simulink model "IEEE_39_IBR_Simplified"  (R2023b)
settings: Solver=FixedStepAuto  StartTime=0  StopTime=20  FixedStep=Ts  MaxStep=1/60  RelTol=1e-3  AbsTol=1e-2  EnableMultiTasking=on
PreLoadFcn:
  | NE39bus_data;
  | PSSMODEL=1;
  | LPSS=0;
  | WAPSS=0;
  | WAPSS2=0;
values from neighbouring files (symbols this model uses):
  Dt = 0    [SG_para.m]
  dw0_sm = 0    [SG_para.m]
  Emax = 1    [SG_para.m]
  Emin = 0.5    [SG_para.m]
  Fg = [0.1,0.1,0.1]    [SG_para.m]
  fn_sm = 60*ones(1,10)    [SG_para.m]
  H_sm = [5,3.03,3.58,2.86,2.6,3.48,2.64,2.43,3.45,4.2]*10    [SG_para.m]
  ia0_sm = 0.75*0    (= 0)    [SG_para.m]
  ib0_sm = 0.75*0    (= 0)    [SG_para.m]
  ic0_sm = 0.75*0    (= 0)    [SG_para.m]
  Kd_sm = 6*ones(1,10)    [SG_para.m]
  Ke = 200    [SG_para.m]
  Kg = [0.95,0.95,0.95]    [SG_para.m]
  Ks = 2    [SG_para.m]
  line = [     1	2	0.0035	0.0411	0.6987	0	100	345 ... (first row only)    [SG_para.m]
  p = 1    [SG_para.m]
  pha0_sm = -24.95*0    (= 0)    [SG_para.m]
  phb0_sm = -144.94*0    (= 0)    [SG_para.m]
  phc0_sm = 95.05*0    (= 0)    [SG_para.m]
  Pn_sm = [1000,1000,1000,1000,1000,1000,1000,1000,1000,1000]    [SG_para.m]
  Pref_sm = [1000 520.81 650 632 508 650 560 540 830 250]./Pn_sm    [SG_para.m]
  R = 1e-3    (= 0.001)    [SG_para.m]
  Rg = [0.05,0.05,0.05]    [SG_para.m]
  rs = 2.8544e-3    (= 0.0028544)    [SG_para.m]
  s = 1    [SG_para.m]
  s1 = 10    [SG_para.m]
  T1 = 0.05    [SG_para.m]
  T2 = 0.5    [SG_para.m]
  T3 = 0.5    [SG_para.m]
  Te = 0.05    [SG_para.m]
  Tfa = 3    [SG_para.m]
  Tfb = 10    [SG_para.m]
  Tg = [10,10,10]    [SG_para.m]
  theta0_sm = -94.3*0    (= 0)    [SG_para.m]
  Ts = 5e-5    (= 5e-05)    [SG_para.m]
  Ts1 = 0.18    [SG_para.m]
  Ts2 = 2    [SG_para.m]
  Ts3 = 5    [SG_para.m]
  Ts4 = 10    [SG_para.m]
  Ts5 = 15    [SG_para.m]
  Un_sm = [345,22,22,22,22,22,22,22,345,22]    [SG_para.m]
  Vmax = inf    [SG_para.m]
  Vmin = 0    [SG_para.m]
  Vref_sm = 1*ones(1,10)    [SG_para.m]
  xd = xd_t    (= 0.296)    [SG_para.m]
undefined symbols (not defined in the file or in its folder): D1, D11, Delta, Ka, Kf, Ta, Tf
libraries: spsThreePhaseVIMeasurementLib x41, spsThreePhaseFaultLib x39, spsThreePhaseSeriesRLCBranchLib x36, spsThreePhaseParallelRLCLoadLib x20, spsThreePhaseTransformerTwoWindingsLib x13, spsSimplifiedSynchronousMachinepuUnitsLib x10, spsLoadFlowBusLib x10, Inverter_based_Resources_IBRs x10, spsThreePhaseBreakerLib x2, spsSequenceAnalyzerLib x2, spsMultimeterLib x1, eePowerMeasurement x1
(part 1 of 5)
settings Model: SimulationMode=accelerator  Creator=Innocent  LastModifiedBy=qholmes
settings SolverCC: AutoScaleAbsTol=off  ZeroCrossAlgorithm=Adaptive  AlgebraicLoopSolver=TrustRegion
settings DataIOCC: SaveFormat=Array  SignalLoggingSaveFormat=ModelDataLogs  SaveOutput=off  SaveTime=off  ReturnWorkspaceOutputs=off
settings OptimizationCC: BlockReduction=off  BooleanDataType=off  ExpressionDepthLimit=2147483647  InitFltsAndDblsToZero=on  LifeSpan=inf
settings DebuggingCC: SaveWithParameterizedLinksMsg=none  UnderspecifiedInitializationDetection=Classic  MergeDetectMultiDrivingBlocksExec=none  SignalResolutionControl=TryResolveAllWithWarning  MaxConsecutiveZCsMsg=none  SolverPrmCheckMsg=warning  MultiTaskDSMMsg=warning  MultiTaskCondExecSysMsg=none  FcnCallInpInsideContextMsg=warning  StateNameClashWarn=warning  SFUnexpectedBacktrackingDiag=warning  SFNoUnconditionalDefaultTransitionDiag=warning  SFExecutionAtInitializationDiag=none  ArithmeticOperatorsInVariantConditions=warning
settings HardwareCC: ProdBitPerPointer=32  ProdBitPerSizeT=32  ProdBitPerPtrDiffT=32  ProdLargestAtomicFloat=None  ProdIntDivRoundTo=Undefined  ProdEndianess=Unspecified  ProdWordSize=32  ProdHWDeviceType=32-bit Generic
settings ModelReferenceCC: EnableRefExpFcnMdlSchedulingChecks=on  PropagateSignalLabelsOutOfModel=off
settings SFSimCC: SimUseLocalCustomCode=off  CustomCodeUndefinedFunction=UseInterfaceOnly
settings RTWCC: RTWUseLocalCustomCode=off  DLArmComputeVersion=19.05
settings CodeAppCC: StateflowObjectComments=on
settings GRTTargetCC: TargetFcnLib=ansi_tfl_tmw.mat  TargetLangStandard=C89/C90 (ANSI)  CombineOutputUpdateFcns=off  GRTInterface=on
settings ConfigComp: CovMetricSettings=dw  CovSaveCumulativeToWorkspaceVar=on  CovSaveSingleToWorkspaceVar=on  CovExternalEMLEnable=off
settings SimscapeCC: SimscapeNormalizeSystem=off

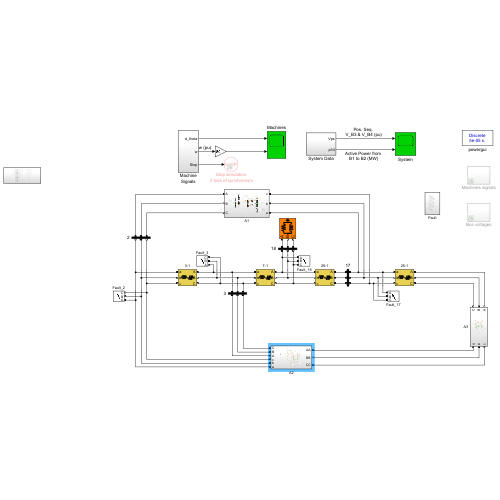
[thumbnail: Simulink's stored preview of the top-level diagram]
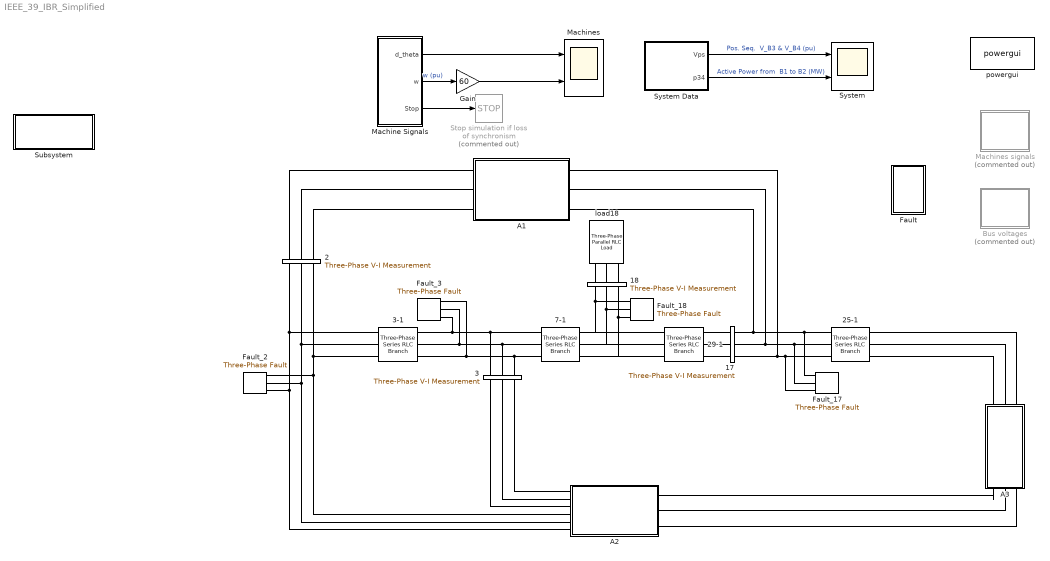
== system IEEE_39_IBR_Simplified ==
  17 : spsThreePhaseVIMeasurementLib/Three-Phase V-I Measurement  VoltageMeasurement=phase-to-phase  SetLabelV=on  LabelV=Vabc_17  Vpu=off  VpuLL=on  CurrentMeasurement=no  SetLabelI=on  LabelI=Iabc_B2  Ipu=off  Pbase=100e6  Vbase=Bus(17,2)*1e3  OutputType=Complex  PhasorSimulation=off  PSBequivalent=0
  18 : spsThreePhaseVIMeasurementLib/Three-Phase V-I Measurement  VoltageMeasurement=phase-to-phase  SetLabelV=on  LabelV=Vabc_18  Vpu=off  VpuLL=on  CurrentMeasurement=no  SetLabelI=on  LabelI=Iabc_B2  Ipu=off  Pbase=100e6  Vbase=Bus(18,2)*1e3  OutputType=Complex  PhasorSimulation=off  PSBequivalent=0
  2 : spsThreePhaseVIMeasurementLib/Three-Phase V-I Measurement  VoltageMeasurement=phase-to-phase  SetLabelV=on  LabelV=Vabc_2  Vpu=off  VpuLL=on  CurrentMeasurement=no  SetLabelI=on  LabelI=Iabc_B2  Ipu=off  Pbase=100e6  Vbase=Bus(2,2)*1e3  OutputType=Complex  PhasorSimulation=off  PSBequivalent=0
  25-1 : spsThreePhaseSeriesRLCBranchLib/Three-Phase Series RLC Branch  LConnTagsString=A|B|C  RConnTagsString=A|B|C  BranchType=RL  Resistance=line(25,3)  Inductance=line(25,4)  Capacitance=1e-6  Measurements=None
  29-1 : spsThreePhaseSeriesRLCBranchLib/Three-Phase Series RLC Branch  LConnTagsString=A|B|C  RConnTagsString=A|B|C  BranchType=RL  Resistance=line(29,3)  Inductance=line(29,4)  Capacitance=1e-6  Measurements=None
  3 : spsThreePhaseVIMeasurementLib/Three-Phase V-I Measurement  VoltageMeasurement=phase-to-phase  SetLabelV=on  LabelV=Vabc_B3  Vpu=off  VpuLL=on  CurrentMeasurement=yes  SetLabelI=on  LabelI=Iabc_B3  Ipu=off  Pbase=100e6  Vbase=Bus(3,2)*1e3  OutputType=Complex  PhasorSimulation=off  PSBequivalent=0
  3-1 : spsThreePhaseSeriesRLCBranchLib/Three-Phase Series RLC Branch  LConnTagsString=A|B|C  RConnTagsString=A|B|C  BranchType=RL  Resistance=line(3,3)  Inductance=line(3,4)  Capacitance=1e-6  Measurements=None
  7-1 : spsThreePhaseSeriesRLCBranchLib/Three-Phase Series RLC Branch  LConnTagsString=A|B|C  RConnTagsString=A|B|C  BranchType=RL  Resistance=line(7,3)  Inductance=line(7,4)  Capacitance=1e-6  Measurements=None
  A1 : Subsystem
  A2 : Subsystem
  A3 : Subsystem
  Bus voltages : Subsystem  Commented=on
  Fault : Subsystem
  Fault_17 : spsThreePhaseFaultLib/Three-Phase Fault  InitialStates=0  FaultA=on  FaultB=on  FaultC=on  GroundFault=on  SwitchTimes="[t(17)+1/60  t(17)+5/60]"  External=off  SwitchStatus=NaN  FaultResistance=0.001  GroundResistance=0.01  SnubberResistance=1e6  SnubberCapacitance=inf  Measurements=Fault voltages and currents
  Fault_18 : spsThreePhaseFaultLib/Three-Phase Fault  InitialStates=0  FaultA=on  FaultB=on  FaultC=on  GroundFault=on  SwitchTimes="[t(18)+1/60  t(18)+5/60]"  External=off  SwitchStatus=NaN  FaultResistance=0.001  GroundResistance=0.01  SnubberResistance=1e6  SnubberCapacitance=inf  Measurements=Fault voltages and currents
  Fault_2 : spsThreePhaseFaultLib/Three-Phase Fault  InitialStates=0  FaultA=on  FaultB=on  FaultC=on  GroundFault=on  SwitchTimes="[t(2)+1/60  t(2)+5/60]"  External=off  SwitchStatus=NaN  FaultResistance=0.001  GroundResistance=0.01  SnubberResistance=1e6  SnubberCapacitance=inf  Measurements=Fault voltages and currents
  Fault_3 : spsThreePhaseFaultLib/Three-Phase Fault  InitialStates=0  FaultA=on  FaultB=on  FaultC=on  GroundFault=on  SwitchTimes="[t(3)+1/60  t(3)+5/60]"  External=off  SwitchStatus=NaN  FaultResistance=0.001  GroundResistance=0.01  SnubberResistance=1e6  SnubberCapacitance=inf  Measurements=Fault voltages and currents
  Gain : Gain  Gain=60
  Machine Signals : Subsystem
  Machines : Scope  NumInputPorts=2
  Machines signals : Subsystem  Commented=on
  Stop simulation if loss of synchronism : Stop  Commented=on
  Subsystem : Subsystem
  System : Scope  NumInputPorts=2
  System Data : Subsystem
  load18 : spsThreePhaseParallelRLCLoadLib/Three-Phase Parallel RLC Load  LConnTagsString=A|B|C  Configuration=Y (grounded)  NominalVoltage=(345000)*0.991132  Vabc=[1e3 1e3 1e3]  Vabcp=[1e3 1e3 1e3]  NominalFrequency=60  UnbalancedPower=off  ActivePower=158e6  InductivePower=30e6  CapacitivePower=0  Pabc=[10e3 9e3 11e3]  QLabc=[100 90 110]  QCabc=[100 90 110]  Pabcp=[10e3 9e3 11e3]  QLabcp=[100 90 110]  QCabcp=[100 90 110]  Measurements=None  LoadType=constant PQ
  powergui : sps_lib/powergui  Priority=2  SimulationMode=Discrete  SampleTime=Ts  frequency=60  Iterations=50  frequencyindice=0  Pbase=100e6  ErrMax=0.0001  UnitsV=kV  UnitsW=MW  buscounter=0  FunctionMessages=off  echomessages=off  EnableUseOfTLC=off  CurrentSourceSwitches=off  DisableSnubberDevices=off  DisableRonSwitches=off  DisableVfSwitches=off  DisplayEquations=off  AutomaticDiscreteSolvers=off  SolverType=Tustin/Backward Euler (TBE)  Interpol=off  ExternalGateDelay=off  methode=off  Ts=100  x0status=blocks  SPID=off  SwTol=0  HookPort=off  NonlinearTolerance=1e-4  nMaxIteration=100  ContinueOnMaxIteration=off  RestoreLinks=warning  ResistiveCurrentMeasurement=off  Frange=logspace(0,3,50)  Ylog=off  Xlog=off  ShowGrid=off  save=off  variable=ZData  structure=0  ZoomFFT=on  StartTime=0.0  cycles=1  DisplayStyle=1  fundamental=60  FreqAxis=off  MaxFrequency=1000  frequencyindicesteady=1  RmsSteady=1  display=off
  wires:
  Machine Signals/2(w) -> Gain/1  "w (pu)"
  Machine Signals/3(Stop) -> Stop simulation if loss of synchronism/1
  Machine Signals/1(d_theta) -> Machines/1
  System Data/1(Vps) -> System/1  "Pos. Seq.  V_B3 & V_B4 (pu)"
  System Data/2(p34) -> System/2  "Active Power from  B1 to B2 (MW)"
  Gain/1 -> Machines/2
  connections:
  29-1/LConn1 -- 17/RConn1
  29-1/LConn2 -- 17/RConn2
  29-1/LConn3 -- 17/RConn3
  load18/LConn1 -- 18/LConn1
  load18/LConn2 -- 18/LConn2
  load18/LConn3 -- 18/LConn3
  3/LConn1 -- 7-1/RConn1 -- 3-1/LConn1 -- Fault_3/LConn1
  Fault_3/LConn2 -- 3-1/LConn2 -- 7-1/RConn2 -- 3/LConn2
  Fault_3/LConn3 -- 3-1/LConn3 -- 7-1/RConn3 -- 3/LConn3
  Fault_2/LConn3 -- A2/LConn4 -- 3-1/RConn3 -- 2/RConn3
  29-1/RConn1 -- 7-1/LConn1 -- Fault_18/LConn1 -- 18/RConn1
  29-1/RConn2 -- 7-1/LConn2 -- Fault_18/LConn2 -- 18/RConn2
  29-1/RConn3 -- 7-1/LConn3 -- Fault_18/LConn3 -- 18/RConn3
  Fault_17/LConn2 -- 25-1/RConn2 -- A1/RConn2 -- 17/LConn2
  Fault_17/LConn3 -- 25-1/RConn3 -- A1/RConn1 -- 17/LConn3
  Fault_17/LConn1 -- 25-1/RConn1 -- A1/RConn3 -- 17/LConn1
  A1/LConn1 -- 2/LConn1
  A1/LConn2 -- 2/LConn2
  A1/LConn3 -- 2/LConn3
  25-1/LConn1 -- A3/LConn3
  25-1/LConn2 -- A3/LConn2
  25-1/LConn3 -- A3/LConn1
  Fault_2/LConn1 -- A2/LConn6 -- 3-1/RConn1 -- 2/RConn1
  Fault_2/LConn2 -- A2/LConn5 -- 3-1/RConn2 -- 2/RConn2
  3/RConn1 -- A2/LConn3
  3/RConn2 -- A2/LConn2
  A2/LConn1 -- 3/RConn3
  A3/RConn1 -- A2/RConn1
  A3/RConn2 -- A2/RConn2
  A3/RConn3 -- A2/RConn3

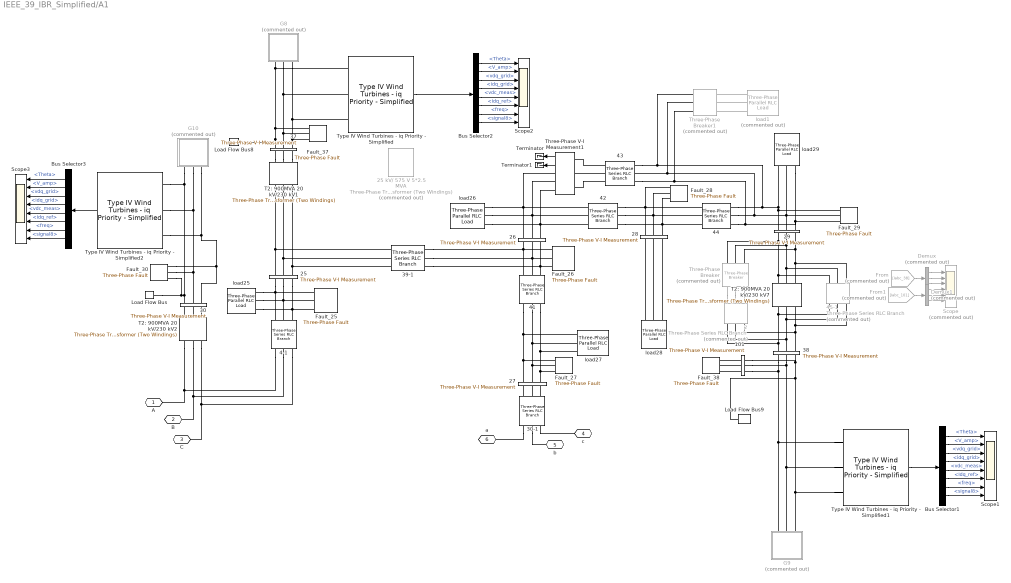
== system IEEE_39_IBR_Simplified/A1 ==
  101 : spsThreePhaseVIMeasurementLib/Three-Phase V-I Measurement  VoltageMeasurement=phase-to-phase  SetLabelV=on  LabelV=Vabc_101  Vpu=off  VpuLL=on  CurrentMeasurement=yes  SetLabelI=on  LabelI=Iabc_101  Ipu=off  Pbase=100e6  Vbase=345*1e3  OutputType=Complex  PhasorSimulation=off  PSBequivalent=0
  2 : spsThreePhaseSeriesRLCBranchLib/Three-Phase Series RLC Branch  Commented=on  LConnTagsString=A|B|C  RConnTagsString=A|B|C  BranchType=RL  Resistance=line(45,3)  Inductance=line(45,4)  Capacitance=1e-6  Measurements=None
  25 : spsThreePhaseVIMeasurementLib/Three-Phase V-I Measurement  VoltageMeasurement=phase-to-phase  SetLabelV=on  LabelV=Vabc_25  Vpu=off  VpuLL=on  CurrentMeasurement=no  SetLabelI=on  LabelI=Iabc_B2  Ipu=off  Pbase=100e6  Vbase=Bus(25,2)*1e3  OutputType=Complex  PhasorSimulation=off  PSBequivalent=0
  25 kV/ 575 V 5*2.5 MVA : spsThreePhaseTransformerTwoWindingsLib/Three-Phase Transformer (Two Windings)  Commented=on  Winding1Connection=Delta (D11)  Winding2Connection=Yg  CoreType=Three single-phase transformers  SetSaturation=off  Hysteresis=off  DataFile='hysteresis'  SetInitialFlux=off  Measurements=None  UNITS=pu  NominalPower="[2.5e6*400  60]"  Winding1=[22e3 , 0.025/30 , 0.025]  Winding2=[ 575, 0.025/30 , 0.025]  Rm=500  Lm=inf  L0=0.5  Saturation=[ 0,0 ; 0.0024,1.2 ; 1.0,1.52 ]  InitialFluxes=[ 0.8 , -0.8 , 0.7 ]  BreakLoop=off  DiscreteSolver=Trapezoidal iterative  DataType=off  TransfoNumber=0
  26 : spsThreePhaseVIMeasurementLib/Three-Phase V-I Measurement  VoltageMeasurement=phase-to-phase  SetLabelV=on  LabelV=Vabc_26  Vpu=off  VpuLL=on  CurrentMeasurement=no  SetLabelI=on  LabelI=Iabc_B2  Ipu=off  Pbase=100e6  Vbase=Bus(26,2)*1e3  OutputType=Complex  PhasorSimulation=off  PSBequivalent=0
  27 : spsThreePhaseVIMeasurementLib/Three-Phase V-I Measurement  VoltageMeasurement=phase-to-phase  SetLabelV=on  LabelV=Vabc_27  Vpu=off  VpuLL=on  CurrentMeasurement=no  SetLabelI=on  LabelI=Iabc_B2  Ipu=off  Pbase=100e6  Vbase=Bus(27,2)*1e3  OutputType=Complex  PhasorSimulation=off  PSBequivalent=0
  28 : spsThreePhaseVIMeasurementLib/Three-Phase V-I Measurement  VoltageMeasurement=phase-to-phase  SetLabelV=on  LabelV=Vabc_28  Vpu=off  VpuLL=on  CurrentMeasurement=no  SetLabelI=on  LabelI=Iabc_B2  Ipu=off  Pbase=100e6  Vbase=Bus(28,2)*1e3  OutputType=Complex  PhasorSimulation=off  PSBequivalent=0
  29 : spsThreePhaseVIMeasurementLib/Three-Phase V-I Measurement  VoltageMeasurement=phase-to-phase  SetLabelV=on  LabelV=Vabc_29  Vpu=off  VpuLL=on  CurrentMeasurement=no  SetLabelI=on  LabelI=Iabc_B2  Ipu=off  Pbase=100e6  Vbase=Bus(29,2)*1e3  OutputType=Complex  PhasorSimulation=off  PSBequivalent=0
  30 : spsThreePhaseVIMeasurementLib/Three-Phase V-I Measurement  VoltageMeasurement=phase-to-phase  SetLabelV=on  LabelV=Vabc_30  Vpu=off  VpuLL=on  CurrentMeasurement=no  SetLabelI=on  LabelI=Iabc_B2  Ipu=off  Pbase=100e6  Vbase=Bus(30,2)*1e3  OutputType=Complex  PhasorSimulation=off  PSBequivalent=0
  30-1 : spsThreePhaseSeriesRLCBranchLib/Three-Phase Series RLC Branch  LConnTagsString=A|B|C  RConnTagsString=A|B|C  BranchType=RL  Resistance=line(30,3)  Inductance=line(30,4)  Capacitance=1e-6  Measurements=None
  37 : spsThreePhaseVIMeasurementLib/Three-Phase V-I Measurement  VoltageMeasurement=phase-to-phase  SetLabelV=on  LabelV=Vabc_37  Vpu=off  VpuLL=on  CurrentMeasurement=no  SetLabelI=on  LabelI=Iabc_B2  Ipu=off  Pbase=100e6  Vbase=Bus(37,2)*1e3  OutputType=Complex  PhasorSimulation=off  PSBequivalent=0
  38 : spsThreePhaseVIMeasurementLib/Three-Phase V-I Measurement  VoltageMeasurement=phase-to-phase  SetLabelV=on  LabelV=Vabc_38  Vpu=off  VpuLL=on  CurrentMeasurement=yes  SetLabelI=on  LabelI=Iabc_38  Ipu=off  Pbase=100e6  Vbase=Bus(38,2)*1e3  OutputType=Complex  PhasorSimulation=off  PSBequivalent=0
  39-1 : spsThreePhaseSeriesRLCBranchLib/Three-Phase Series RLC Branch  LConnTagsString=A|B|C  RConnTagsString=A|B|C  BranchType=RL  Resistance=0  Inductance=0.001  Capacitance=1e-6  Measurements=None
  4-1 : spsThreePhaseSeriesRLCBranchLib/Three-Phase Series RLC Branch  LConnTagsString=A|B|C  RConnTagsString=A|B|C  BranchType=RL  Resistance=line(4,3)  Inductance=line(4,4)  Capacitance=1e-6  Measurements=None
  41 : spsThreePhaseSeriesRLCBranchLib/Three-Phase Series RLC Branch  LConnTagsString=A|B|C  RConnTagsString=A|B|C  BranchType=RL  Resistance=line(41,3)  Inductance=line(41,4)  Capacitance=1e-6  Measurements=None
  42 : spsThreePhaseSeriesRLCBranchLib/Three-Phase Series RLC Branch  LConnTagsString=A|B|C  RConnTagsString=A|B|C  BranchType=RL  Resistance=line(42,3)  Inductance=line(42,4)  Capacitance=1e-6  Measurements=None
  43 : spsThreePhaseSeriesRLCBranchLib/Three-Phase Series RLC Branch  LConnTagsString=A|B|C  RConnTagsString=A|B|C  BranchType=RL  Resistance=line(43,3)  Inductance=line(43,4)  Capacitance=1e-6  Measurements=None
  44 : spsThreePhaseSeriesRLCBranchLib/Three-Phase Series RLC Branch  LConnTagsString=A|B|C  RConnTagsString=A|B|C  BranchType=RL  Resistance=line(44,3)  Inductance=line(44,4)  Capacitance=1e-6  Measurements=None
  45-1 : spsThreePhaseSeriesRLCBranchLib/Three-Phase Series RLC Branch  Commented=on  LConnTagsString=A|B|C  RConnTagsString=A|B|C  BranchType=RL  Resistance=line(45,3)  Inductance=0.3*10  Capacitance=1e-6  Measurements=None
  Bus Selector1 : BusSelector  OutputSignals=Theta,V_amp,vdq_grid,idq_grid,vdc_meas,Idq_ref,freq,signal8
  Bus Selector2 : BusSelector  OutputSignals=Theta,V_amp,vdq_grid,idq_grid,vdc_meas,Idq_ref,freq,signal8
  Bus Selector3 : BusSelector  OutputSignals=Theta,V_amp,vdq_grid,idq_grid,vdc_meas,Idq_ref,freq,signal8
  Demux : Demux  Commented=on  Outputs=3
  Demux1 : Demux  Commented=on  Outputs=3
  Fault_25 : spsThreePhaseFaultLib/Three-Phase Fault  InitialStates=0  FaultA=on  FaultB=on  FaultC=on  GroundFault=on  SwitchTimes="[t(25)+1/60  t(25)+5/60]"  External=off  SwitchStatus=NaN  FaultResistance=0.001  GroundResistance=0.01  SnubberResistance=1e6  SnubberCapacitance=inf  Measurements=Fault voltages and currents
  Fault_26 : spsThreePhaseFaultLib/Three-Phase Fault  InitialStates=0  FaultA=on  FaultB=on  FaultC=on  GroundFault=on  SwitchTimes="[t(26)+1/60  t(26)+5/60]"  External=off  SwitchStatus=NaN  FaultResistance=0.001  GroundResistance=0.01  SnubberResistance=1e6  SnubberCapacitance=inf  Measurements=Fault voltages and currents
  Fault_27 : spsThreePhaseFaultLib/Three-Phase Fault  InitialStates=0  FaultA=on  FaultB=on  FaultC=on  GroundFault=on  SwitchTimes="[t(27)+1/60  t(27)+5/60]"  External=off  SwitchStatus=NaN  FaultResistance=0.001  GroundResistance=0.01  SnubberResistance=1e6  SnubberCapacitance=inf  Measurements=Fault voltages and currents
  Fault_28 : spsThreePhaseFaultLib/Three-Phase Fault  InitialStates=0  FaultA=on  FaultB=on  FaultC=on  GroundFault=on  SwitchTimes="[t(28)+1/60  t(28)+5/60]"  External=off  SwitchStatus=NaN  FaultResistance=0.001  GroundResistance=0.01  SnubberResistance=1e6  SnubberCapacitance=inf  Measurements=Fault voltages and currents
  Fault_29 : spsThreePhaseFaultLib/Three-Phase Fault  InitialStates=0  FaultA=on  FaultB=on  FaultC=on  GroundFault=on  SwitchTimes="[t(29)+1/60  t(29)+5/60]"  External=off  SwitchStatus=NaN  FaultResistance=0.001  GroundResistance=0.01  SnubberResistance=1e6  SnubberCapacitance=inf  Measurements=Fault voltages and currents
  Fault_30 : spsThreePhaseFaultLib/Three-Phase Fault  InitialStates=0  FaultA=on  FaultB=on  FaultC=on  GroundFault=on  SwitchTimes="[t(30)+1/60  t(30)+5/60]"  External=off  SwitchStatus=NaN  FaultResistance=0.001  GroundResistance=0.01  SnubberResistance=1e6  SnubberCapacitance=inf  Measurements=Fault voltages and currents
  Fault_37 : spsThreePhaseFaultLib/Three-Phase Fault  InitialStates=0  FaultA=on  FaultB=on  FaultC=on  GroundFault=on  SwitchTimes="[t(37)+1/60  t(37)+5/60]"  External=off  SwitchStatus=NaN  FaultResistance=0.001  GroundResistance=0.01  SnubberResistance=1e6  SnubberCapacitance=inf  Measurements=Fault voltages and currents
  Fault_38 : spsThreePhaseFaultLib/Three-Phase Fault  InitialStates=0  FaultA=on  FaultB=on  FaultC=on  GroundFault=on  SwitchTimes="[t(38)+1/60  t(38)+5/60]"  External=off  SwitchStatus=NaN  FaultResistance=0.001  GroundResistance=0.01  SnubberResistance=1e6  SnubberCapacitance=inf  Measurements=Fault voltages and currents
  From : From  Commented=on  GotoTag=Iabc_38  TagVisibility=global
  From1 : From  Commented=on  GotoTag=Iabc_101  TagVisibility=global
  G10 : Subsystem  Commented=on
  G8 : Subsystem  Commented=on
  G9 : Subsystem  Commented=on
  Load Flow Bus : spsLoadFlowBusLib/Load Flow Bus  LConnTagsString=a  Phases=single  Connectors=on one side  ID=B30  Vbase=22e3  Vref=1.0475  Vangle=0  VLF=1.048  VLFb=1  VLFc=1  angleLF=-3.646  angleLFb=0  angleLFc=0
      settings: AttributesFormatString=%<ID>\n%<Vbase>\n%<VLF>pu\n%<angleLF>deg.
  Load Flow Bus8 : spsLoadFlowBusLib/Load Flow Bus  LConnTagsString=a  Phases=single  Connectors=on one side  ID=Bus37  Vbase=22e3  Vref=1.0278  Vangle=0  VLF=1.028  VLFb=1  VLFc=1  angleLF=2.181  angleLFb=0  angleLFc=0
      settings: AttributesFormatString=%<ID>\n%<Vbase>V\n%<VLF>pu\n%<angleLF>deg.
  Load Flow Bus9 : spsLoadFlowBusLib/Load Flow Bus  LConnTagsString=a  Phases=single  Connectors=on one side  ID=Bus38  Vbase=22e3  Vref=1.0265  Vangle=0  VLF=1.027  VLFb=1  VLFc=1  angleLF=7.784  angleLFb=0  angleLFc=0
      settings: AttributesFormatString=%<ID>\n%<Vbase>V\n%<VLF>pu\n%<angleLF>deg.
  Scope : Scope  Commented=on  NumInputPorts=6
  Scope1 : Scope  NumInputPorts=8
  Scope2 : Scope  NumInputPorts=8
  Scope3 : Scope  NumInputPorts=8
  T2: 900MVA 20 kV/230 kV1 : spsThreePhaseTransformerTwoWindingsLib/Three-Phase Transformer (Two Windings)  Winding1Connection=Delta (D1)  Winding2Connection=Yg  CoreType=Three single-phase transformers  SetSaturation=off  Hysteresis=off  DataFile='hysteresis'  SetInitialFlux=off  Measurements=None  UNITS=pu  NominalPower=[ 1000e6 60 ]  Winding1="[ 22e3 0.0003*s  0]"  Winding2="[ 345e3*1.0 0.0003*s  0.0232*s]"  Rm=500  Lm=500  L0=0.5  Saturation="[ 0,0  ;  0.005,1.2  ;  1.0,1.4 ]"  InitialFluxes=[ 0.8 , -0.8 , 0.7 ]  BreakLoop=off  DiscreteSolver=Trapezoidal iterative  DataType=off  TransfoNumber=0
  T2: 900MVA 20 kV/230 kV2 : spsThreePhaseTransformerTwoWindingsLib/Three-Phase Transformer (Two Windings)  Winding1Connection=Delta (D1)  Winding2Connection=Yg  CoreType=Three single-phase transformers  SetSaturation=off  Hysteresis=off  DataFile='hysteresis'  SetInitialFlux=off  Measurements=None  UNITS=pu  NominalPower=[ 1000e6 60 ]  Winding1="[ 22e3*1.0  1e-6  0]"  Winding2="[ 345e3*1.0  1e-6  0.0181*s]"  Rm=500  Lm=500  L0=0.5  Saturation="[ 0,0  ;  0.005,1.2  ;  1.0,1.4 ]"  InitialFluxes=[ 0.8 , -0.8 , 0.7 ]  BreakLoop=off  DiscreteSolver=Trapezoidal iterative  DataType=off  TransfoNumber=0
  T2: 900MVA 20 kV/230 kV7 : spsThreePhaseTransformerTwoWindingsLib/Three-Phase Transformer (Two Windings)  Winding1Connection=Delta (D1)  Winding2Connection=Yg  CoreType=Three single-phase transformers  SetSaturation=off  Hysteresis=off  DataFile='hysteresis'  SetInitialFlux=off  Measurements=None  UNITS=pu  NominalPower=[ 1000e6 60 ]  Winding1="[345e3*1.  0.0004*s  0]"  Winding2="[ 345e3*1.0  0.0004*s  0.0156*s]"  Rm=500  Lm=500  L0=0.5  Saturation="[ 0,0  ;  0.005,1.2  ;  1.0,1.4 ]"  InitialFluxes=[ 0.8 , -0.8 , 0.7 ]  BreakLoop=off  DiscreteSolver=Trapezoidal iterative  DataType=off  TransfoNumber=0
  Terminator : Terminator
  Terminator1 : Terminator
  Three-Phase V-I Measurement1 : spsThreePhaseVIMeasurementLib/Three-Phase V-I Measurement  VoltageMeasurement=phase-to-ground  SetLabelV=off  LabelV=Vabc  Vpu=off  VpuLL=off  CurrentMeasurement=yes  SetLabelI=off  LabelI=Iabc  Ipu=off  Pbase=100e6  Vbase=500e3  OutputType=Complex  PhasorSimulation=off  PSBequivalent=0
  Three-Phase Breaker : spsThreePhaseBreakerLib/Three-Phase Breaker  Commented=on  InitialState=closed  SwitchA=on  SwitchB=on  SwitchC=on  SwitchTimes=[120, 130]  External=off  BreakerResistance=0.01  SnubberResistance=1e6  SnubberCapacitance=inf  Measurements=None
  Three-Phase Breaker1 : spsThreePhaseBreakerLib/Three-Phase Breaker  Commented=on  InitialState=open  SwitchA=on  SwitchB=on  SwitchC=on  SwitchTimes=30  External=off  BreakerResistance=0.01  SnubberResistance=1e6  SnubberCapacitance=inf  Measurements=None
  Type IV Wind Turbines - iq Priority - Simplified : Inverter_based_Resources_IBRs/Inverter-based Resources (IBRs)/Type IV Wind Turbines - iq Priority - Simplified  Num_WTs=1  Wind_Speed_WT=15  Q_ref_pu_WT=0  Transformer_P_f="[1000e6  60]"  Transformer_V1_R1_L1=[22e3 , 0.025/30 , 0.025]  DC_Power=1000e6*0.3986
  Type IV Wind Turbines - iq Priority - Simplified1 : Inverter_based_Resources_IBRs/Inverter-based Resources (IBRs)/Type IV Wind Turbines - iq Priority - Simplified  Num_WTs=1  Wind_Speed_WT=15  Q_ref_pu_WT=0  Transformer_P_f="[1000e6  60]"  Transformer_V1_R1_L1=[345e3 , 0.025/30 , 0.025]  DC_Power=1000e6*0.6893
  Type IV Wind Turbines - iq Priority - Simplified2 : Inverter_based_Resources_IBRs/Inverter-based Resources (IBRs)/Type IV Wind Turbines - iq Priority - Simplified  Num_WTs=1  Wind_Speed_WT=15  Q_ref_pu_WT=0  Transformer_P_f="[1000e6  60]"  Transformer_V1_R1_L1=[22e3 , 0.025/30 , 0.025]  DC_Power=1000e6*0.1093
  load1 : spsThreePhaseParallelRLCLoadLib/Three-Phase Parallel RLC Load  Commented=on  LConnTagsString=A|B|C  Configuration=Y (grounded)  NominalVoltage=(345000)*1.02077  Vabc=[1e3 1e3 1e3]  Vabcp=[1e3 1e3 1e3]  NominalFrequency=60  UnbalancedPower=off  ActivePower=383.5e6  InductivePower=26.9e6  CapacitivePower=0  Pabc=[10e3 9e3 11e3]  QLabc=[100 90 110]  QCabc=[100 90 110]  Pabcp=[10e3 9e3 11e3]  QLabcp=[100 90 110]  QCabcp=[100 90 110]  Measurements=None  LoadType=constant PQ
  load25 : spsThreePhaseParallelRLCLoadLib/Three-Phase Parallel RLC Load  LConnTagsString=A|B|C  Configuration=Y (grounded)  NominalVoltage=(345000)*1.0284  Vabc=[1e3 1e3 1e3]  Vabcp=[1e3 1e3 1e3]  NominalFrequency=60  UnbalancedPower=off  ActivePower=224e6  InductivePower=47.2e6  CapacitivePower=0  Pabc=[10e3 9e3 11e3]  QLabc=[100 90 110]  QCabc=[100 90 110]  Pabcp=[10e3 9e3 11e3]  QLabcp=[100 90 110]  QCabcp=[100 90 110]  Measurements=None  LoadType=constant PQ
  load26 : spsThreePhaseParallelRLCLoadLib/Three-Phase Parallel RLC Load  LConnTagsString=A|B|C  Configuration=Y (grounded)  NominalVoltage=(345000)*1.01809  Vabc=[1e3 1e3 1e3]  Vabcp=[1e3 1e3 1e3]  NominalFrequency=60  UnbalancedPower=off  ActivePower=539e6/539*139  InductivePower=17e6  CapacitivePower=0  Pabc=[10e3 9e3 11e3]  QLabc=[100 90 110]  QCabc=[100 90 110]  Pabcp=[10e3 9e3 11e3]  QLabcp=[100 90 110]  QCabcp=[100 90 110]  Measurements=None  LoadType=constant PQ
  load27 : spsThreePhaseParallelRLCLoadLib/Three-Phase Parallel RLC Load  LConnTagsString=A|B|C  Configuration=Y (grounded)  NominalVoltage=(345000)*1.00029  Vabc=[1e3 1e3 1e3]  Vabcp=[1e3 1e3 1e3]  NominalFrequency=60  UnbalancedPower=off  ActivePower=281e6  InductivePower=75.5e6  CapacitivePower=0  Pabc=[10e3 9e3 11e3]  QLabc=[100 90 110]  QCabc=[100 90 110]  Pabcp=[10e3 9e3 11e3]  QLabcp=[100 90 110]  QCabcp=[100 90 110]  Measurements=None  LoadType=constant PQ
  load28 : spsThreePhaseParallelRLCLoadLib/Three-Phase Parallel RLC Load  LConnTagsString=A|B|C  Configuration=Y (grounded)  NominalVoltage=(345000)*1.01937  Vabc=[1e3 1e3 1e3]  Vabcp=[1e3 1e3 1e3]  NominalFrequency=60  UnbalancedPower=off  ActivePower=206e6  InductivePower=27.6e6  CapacitivePower=0  Pabc=[10e3 9e3 11e3]  QLabc=[100 90 110]  QCabc=[100 90 110]  Pabcp=[10e3 9e3 11e3]  QLabcp=[100 90 110]  QCabcp=[100 90 110]  Measurements=None  LoadType=constant PQ
  load29 : spsThreePhaseParallelRLCLoadLib/Three-Phase Parallel RLC Load  LConnTagsString=A|B|C  Configuration=Y (grounded)  NominalVoltage=(345000)*1.02077  Vabc=[1e3 1e3 1e3]  Vabcp=[1e3 1e3 1e3]  NominalFrequency=60  UnbalancedPower=off  ActivePower=283.5e6  InductivePower=26.9e6  CapacitivePower=0  Pabc=[10e3 9e3 11e3]  QLabc=[100 90 110]  QCabc=[100 90 110]  Pabcp=[10e3 9e3 11e3]  QLabcp=[100 90 110]  QCabcp=[100 90 110]  Measurements=None  LoadType=constant PQ
  A : PMIOPort  Side=Left
  B : PMIOPort  Port=2  Side=Left
  C : PMIOPort  Port=3  Side=Left
  c : PMIOPort  Port=4  Side=Right
  b : PMIOPort  Port=5  Side=Right
  a : PMIOPort  Port=6  Side=Right
  wires:
  Three-Phase V-I Measurement1/2 -> Terminator1/1
  Three-Phase V-I Measurement1/1 -> Terminator/1
  From/1 -> Demux/1
  Demux/1 -> Scope/1
  Demux/2 -> Scope/2
  Demux/3 -> Scope/3
  Demux1/2 -> Scope/5
  From1/1 -> Demux1/1
  Demux1/3 -> Scope/6
  Demux1/1 -> Scope/4
  Bus Selector2/3 -> Scope2/3  "<vdq_grid>"
  Bus Selector2/8 -> Scope2/8  "<signal8>"
  Type IV Wind Turbines - iq Priority - Simplified/1 -> Bus Selector2/1
  Bus Selector2/6 -> Scope2/6  "<Idq_ref>"
  Bus Selector2/4 -> Scope2/4  "<idq_grid>"
  Bus Selector2/1 -> Scope2/1  "<Theta>"
  Bus Selector2/7 -> Scope2/7  "<freq>"
  Bus Selector2/2 -> Scope2/2  "<V_amp>"
  Bus Selector2/5 -> Scope2/5  "<vdc_meas>"
  Bus Selector1/3 -> Scope1/3  "<vdq_grid>"
  Bus Selector1/2 -> Scope1/2  "<V_amp>"
  Bus Selector1/4 -> Scope1/4  "<idq_grid>"
  Bus Selector1/5 -> Scope1/5  "<vdc_meas>"
  Bus Selector1/6 -> Scope1/6  "<Idq_ref>"
  Bus Selector1/1 -> Scope1/1  "<Theta>"
  Bus Selector1/8 -> Scope1/8  "<signal8>"
  Type IV Wind Turbines - iq Priority - Simplified1/1 -> Bus Selector1/1
  Bus Selector1/7 -> Scope1/7  "<freq>"
  Bus Selector3/3 -> Scope3/3  "<vdq_grid>"
  Bus Selector3/2 -> Scope3/2  "<V_amp>"
  Bus Selector3/4 -> Scope3/4  "<idq_grid>"
  Bus Selector3/5 -> Scope3/5  "<vdc_meas>"
  Bus Selector3/6 -> Scope3/6  "<Idq_ref>"
  Bus Selector3/1 -> Scope3/1  "<Theta>"
  Bus Selector3/8 -> Scope3/8  "<signal8>"
  Type IV Wind Turbines - iq Priority - Simplified2/1 -> Bus Selector3/1
  Bus Selector3/7 -> Scope3/7  "<freq>"
  connections:
  Fault_28/LConn3 -- 44/RConn3 -- 42/LConn3 -- 28/RConn3
  29/RConn1 -- Three-Phase Breaker1/LConn1 -- 43/LConn1 -- 44/LConn1 -- load29/LConn1 -- Fault_29/LConn1
  43/RConn3 -- Three-Phase V-I Measurement1/LConn3
  Fault_25/LConn1 -- 4-1/LConn1 -- 25/RConn1 -- load25/LConn1
  43/RConn1 -- Three-Phase V-I Measurement1/LConn1
  T2: 900MVA 20 kV/230 kV2/RConn3 -- C/RConn1 -- 4-1/RConn3
  30/LConn3 -- Type IV Wind Turbines - iq Priority - Simplified2/LConn3 -- G10/LConn3 -- Fault_30/LConn3
  load27/LConn1 -- 27/LConn1 -- Fault_27/LConn1 -- 41/RConn1
  T2: 900MVA 20 kV/230 kV2/RConn1 -- A/RConn1 -- 4-1/RConn1
  29/RConn2 -- load29/LConn2 -- Fault_29/LConn2 -- 44/LConn2 -- Three-Phase Breaker1/LConn2 -- 43/LConn2
  30-1/LConn3 -- 27/RConn3
  28/RConn1 -- 44/RConn1 -- 42/LConn1 -- Fault_28/LConn1
  T2: 900MVA 20 kV/230 kV7/LConn3 -- 45-1/LConn3 -- 2/LConn3 -- 38/LConn3
  T2: 900MVA 20 kV/230 kV2/RConn2 -- B/RConn1 -- 4-1/RConn2
  30/RConn1 -- T2: 900MVA 20 kV/230 kV2/LConn1
  T2: 900MVA 20 kV/230 kV7/LConn1 -- 45-1/LConn1 -- 2/LConn1 -- 38/LConn1
  Fault_25/LConn3 -- 25/RConn3 -- 4-1/LConn3 -- load25/LConn3
  30-1/RConn2 -- b/RConn1
  39-1/LConn1 -- 25/LConn1 -- T2: 900MVA 20 kV/230 kV1/RConn1
  26/RConn3 -- 39-1/RConn3 -- 41/LConn3 -- Fault_26/LConn3
  30-1/RConn3 -- c/RConn1
  load27/LConn3 -- 27/LConn3 -- Fault_27/LConn3 -- 41/RConn3
  Fault_25/LConn2 -- 4-1/LConn2 -- 25/RConn2 -- load25/LConn2
  38/RConn1 -- 101/RConn1 -- G9/LConn1 -- Type IV Wind Turbines - iq Priority - Simplified1/LConn1
  T2: 900MVA 20 kV/230 kV7/RConn3 -- 45-1/RConn3 -- Three-Phase Breaker/RConn3 -- 29/LConn3
  26/RConn2 -- 39-1/RConn2 -- 41/LConn2 -- Fault_26/LConn2
  38/RConn3 -- Load Flow Bus9/LConn1 -- G9/LConn3 -- Type IV Wind Turbines - iq Priority - Simplified1/LConn3 -- 101/RConn3
  37/LConn3 -- G8/LConn3 -- Type IV Wind Turbines - iq Priority - Simplified/LConn3 -- Fault_37/LConn3
  Three-Phase V-I Measurement1/RConn1 -- 26/LConn1 -- 42/RConn1 -- load26/LConn1
  37/RConn2 -- T2: 900MVA 20 kV/230 kV1/LConn2
  Three-Phase V-I Measurement1/RConn3 -- 26/LConn3 -- 42/RConn3 -- load26/LConn3
  29/LConn2 -- Three-Phase Breaker/RConn2 -- 45-1/RConn2 -- T2: 900MVA 20 kV/230 kV7/RConn2
  Three-Phase V-I Measurement1/RConn2 -- 26/LConn2 -- 42/RConn2 -- load26/LConn2
  30/LConn1 -- Type IV Wind Turbines - iq Priority - Simplified2/LConn1 -- G10/LConn1 -- Load Flow Bus/LConn1 -- Fault_30/LConn1
  26/RConn1 -- 39-1/RConn1 -- 41/LConn1 -- Fault_26/LConn1
  30/RConn3 -- T2: 900MVA 20 kV/230 kV2/LConn3
  30/LConn2 -- Type IV Wind Turbines - iq Priority - Simplified2/LConn2 -- G10/LConn2 -- Fault_30/LConn2
  38/RConn2 -- 101/RConn2 -- G9/LConn2 -- Type IV Wind Turbines - iq Priority - Simplified1/LConn2
  load27/LConn2 -- 27/LConn2 -- Fault_27/LConn2 -- 41/RConn2
  39-1/LConn2 -- 25/LConn2 -- T2: 900MVA 20 kV/230 kV1/RConn2
  T2: 900MVA 20 kV/230 kV7/LConn2 -- 45-1/LConn2 -- 2/LConn2 -- 38/LConn2
  28/RConn2 -- 44/RConn2 -- 42/LConn2 -- Fault_28/LConn2
  load29/LConn3 -- Fault_29/LConn3 -- Three-Phase Breaker1/LConn3 -- 43/LConn3 -- 44/LConn3 -- 29/RConn3
  30-1/LConn2 -- 27/RConn2
  43/RConn2 -- Three-Phase V-I Measurement1/LConn2
  37/LConn2 -- G8/LConn2 -- Type IV Wind Turbines - iq Priority - Simplified/LConn2 -- Fault_37/LConn2
  30/RConn2 -- T2: 900MVA 20 kV/230 kV2/LConn2
  30-1/RConn1 -- a/RConn1
  T2: 900MVA 20 kV/230 kV1/RConn3 -- 25/LConn3 -- 39-1/LConn3
  37/RConn3 -- T2: 900MVA 20 kV/230 kV1/LConn3
  load28/LConn2 -- 28/LConn2
  T2: 900MVA 20 kV/230 kV7/RConn1 -- Three-Phase Breaker/RConn1 -- 29/LConn1 -- 45-1/RConn1
  37/RConn1 -- T2: 900MVA 20 kV/230 kV1/LConn1
  load28/LConn1 -- 28/LConn1
  load28/LConn3 -- 28/LConn3
  30-1/LConn1 -- 27/RConn1
  Three-Phase Breaker/LConn1 -- 2/RConn1
  Three-Phase Breaker/LConn2 -- 2/RConn2
  Three-Phase Breaker/LConn3 -- 2/RConn3
  load1/LConn1 -- Three-Phase Breaker1/RConn1
  load1/LConn2 -- Three-Phase Breaker1/RConn2
  load1/LConn3 -- Three-Phase Breaker1/RConn3
  101/LConn1 -- Fault_38/LConn1
  101/LConn2 -- Fault_38/LConn2
  101/LConn3 -- Fault_38/LConn3
  37/LConn1 -- Load Flow Bus8/LConn1 -- G8/LConn1 -- Type IV Wind Turbines - iq Priority - Simplified/LConn1 -- Fault_37/LConn1
